simulink model "TD4_Ex_sim_part1_1"  (R2022a)
settings: Solver=VariableStepAuto  StartTime=0.0  StopTime=20  RelTol=1e-3
undefined symbols (not defined in the file): A_obs, B_obs, C_obs, D_obs, K, l, N, xinit_obs
settings Model: Creator=CS  LastModifiedBy=CS

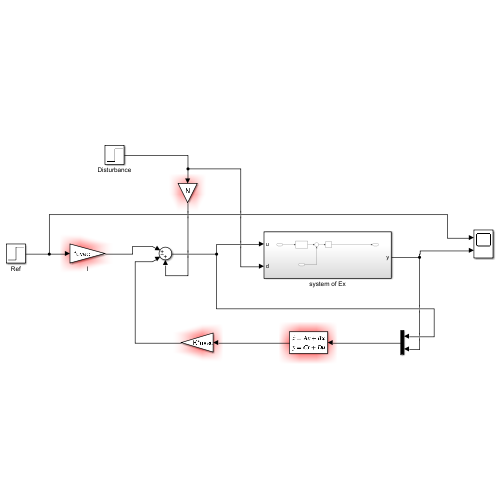
[thumbnail: Simulink's stored preview of the top-level diagram]
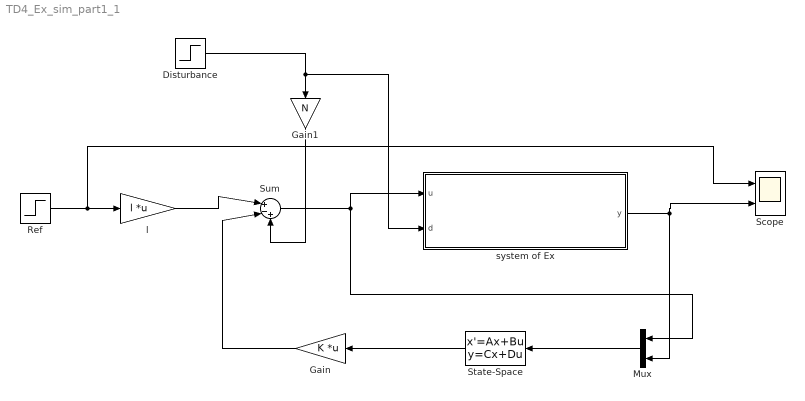
== system TD4_Ex_sim_part1_1 ==
  Disturbance : Step  Time=10  SampleTime=0
  Gain : Gain  Gain=K  Multiplication=Matrix(K*u) (u vector)
  Gain1 : Gain  Gain=N
  Mux : Mux  Inputs=2
  Ref : Step  Time=5  SampleTime=0
  Scope : Scope  NumInputPorts=2
  State-Space : StateSpace  A=A_obs  B=B_obs  C=C_obs  D=D_obs  InitialCondition=xinit_obs
  Sum : Sum  Inputs=|+-+
  l : Gain  Gain=l  Multiplication=Matrix(K*u) (u vector)
  system of Ex : Subsystem
  wires:
  Sum/1 -> Mux/1, system of Ex/1(u)
  system of Ex/1(y) -> Mux/2, Scope/2
  l/1 -> Sum/1
  Gain/1 -> Sum/2
  Ref/1 -> l/1, Scope/1
  Mux/1 -> State-Space/1
  State-Space/1 -> Gain/1
  Disturbance/1 -> system of Ex/2(d), Gain1/1
  Gain1/1 -> Sum/3

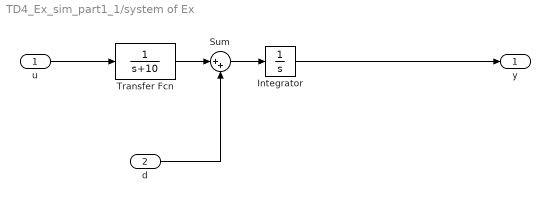
== system TD4_Ex_sim_part1_1/system of Ex ==
  u : Inport
  d : Inport  Port=2
  Integrator : Integrator
  Sum : Sum  Inputs=|++
  Transfer Fcn : TransferFcn  Denominator=[1 10]
  y : Outport
  wires:
  u/1 -> Transfer Fcn/1
  Integrator/1 -> y/1
  Transfer Fcn/1 -> Sum/1
  d/1 -> Sum/2
  Sum/1 -> Integrator/1
